simulink model "maglev_nonlinear"  (R2024a)
settings: Solver=VariableStepAuto  StartTime=0.0  StopTime=tsim  RelTol=1e-3
values from neighbouring files (symbols this model uses):
  cden = den{:}    [sim_maglev.m]
  cnum = num{:}    [sim_maglev.m]
  ref = 0.025+0.001    (= 0.026)    [sim_maglev.m]
  us = 3.39 * is    [sim_maglev.m]
  xs = [is, ys, 0]    [sim_maglev.m]
settings Model: Creator=Meenakshi Mahagaokar  LastModifiedBy=Meenakshi Mahagaokar
settings DataIOCC: SaveOutput=off  DSMLogging=off  SaveTime=off  ReturnWorkspaceOutputs=off

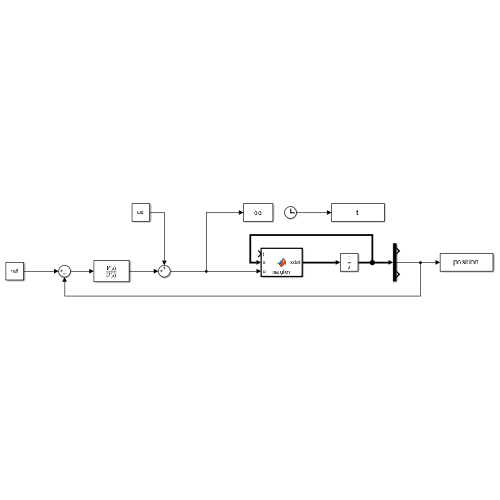
[thumbnail: Simulink's stored preview of the top-level diagram]
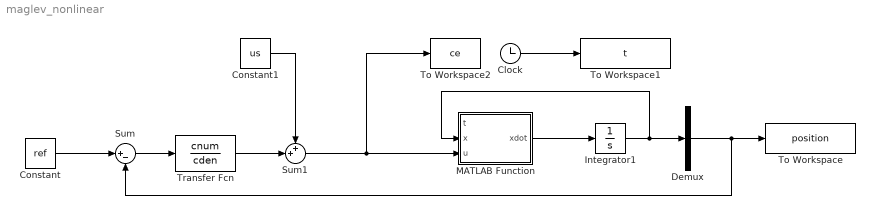
== system maglev_nonlinear ==
  Clock : Clock
  Constant : Constant  Value=ref
  Constant1 : Constant  Value=us
  Demux : Demux  Outputs=3
  Integrator1 : Integrator  InitialCondition=xs
  MATLAB Function : MATLAB Function  TreatAsAtomicUnit=on
  Sum : Sum  Inputs=|+-
  Sum1 : Sum  Inputs=++|
  To Workspace : ToWorkspace  VariableName=position  SampleTime=-1
      settings: Save2DSignal=2-D array (concatenate along first dimension)
  To Workspace1 : ToWorkspace  VariableName=t  SampleTime=-1
      settings: Save2DSignal=2-D array (concatenate along first dimension)
  To Workspace2 : ToWorkspace  VariableName=ce  SampleTime=-1
      settings: Save2DSignal=2-D array (concatenate along first dimension)
  Transfer Fcn : TransferFcn  Numerator=cnum  Denominator=cden
  wires:
  Clock/1 -> To Workspace1/1
  Constant/1 -> Sum/1
  MATLAB Function/1(xdot) -> Integrator1/1
  Integrator1/1 -> MATLAB Function/2(x), Demux/1
  Constant1/1 -> Sum1/1
  Sum/1 -> Transfer Fcn/1
  Transfer Fcn/1 -> Sum1/2
  Demux/2 -> To Workspace/1, Sum/2
  Sum1/1 -> MATLAB Function/3(u), To Workspace2/1

== matlab function maglev_nonlinear/MATLAB Function ==
  data: t input; x input; u input; xdot output
function xdot = maglev(t, x, u)

xdot = maglev(t, x, u);
